simulink model "LQR_SHUM"  (R2015a)
settings: Solver=ode45  StartTime=0.0  StopTime=20  RelTol=1e-3
values from neighbouring files (symbols this model uses):
  Ki = -Kp1(:,1:2)    [Sc_LQR.m]
  Kp = Kp1(:,3:6)    [Sc_LQR.m]
undefined symbols (not defined in the file or in its folder): A, B, C
settings Model: CovSFcnEnable=off  Creator=jordan  LastModifiedBy=Vladislav
settings DebuggingCC: SolverPrmCheckMsg=warning

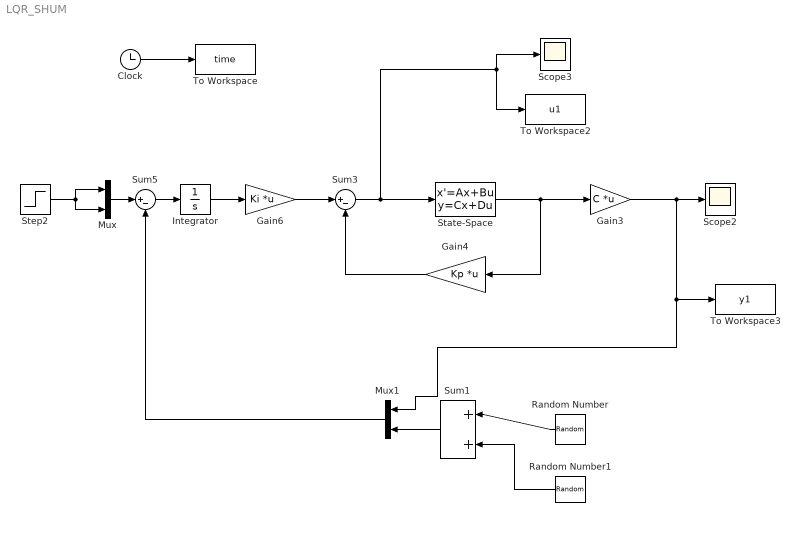
== system LQR_SHUM ==
  Clock : Clock
  Gain3 : Gain  Gain=C  Multiplication=Matrix(K*u)
  Gain4 : Gain  Gain=Kp  Multiplication=Matrix(K*u)
  Gain6 : Gain  Gain=Ki  Multiplication=Matrix(K*u)
  Integrator : Integrator
  Mux : Mux  Inputs=2
  Mux1 : Mux  Inputs=2
  Random Number : RandomNumber  Variance=0.1  SampleTime=0.1
  Random Number1 : RandomNumber  Variance=0.1  Seed=1  SampleTime=0.1
  Scope2 : Scope
      settings: TimeRange=10  YMin=-0.2  YMax=1.4  SaveName=ScopeData2
  Scope3 : Scope
      settings: TimeRange=10  YMin=-0.2  YMax=1.4  SaveName=ScopeData3
  State-Space : StateSpace  A=A  B=B  C=eye(4)  D=zeros(4,2)  X0=0
  Step2 : Step  Time=0  SampleTime=0
  Sum1 : Sum  Inputs=|++
  Sum3 : Sum  Inputs=|+-
  Sum5 : Sum  Inputs=|+-
  To Workspace : ToWorkspace  VariableName=time  SampleTime=-1
  To Workspace2 : ToWorkspace  VariableName=u1  SampleTime=-1
  To Workspace3 : ToWorkspace  VariableName=y1  SampleTime=-1
  wires:
  Sum3/1 -> State-Space/1, To Workspace2/1, Scope3/1
  Gain4/1 -> Sum3/2
  State-Space/1 -> Gain3/1, Gain4/1
  Integrator/1 -> Gain6/1
  Gain6/1 -> Sum3/1
  Step2/1 -> Mux/1, Mux/2
  Mux/1 -> Sum5/1
  Sum5/1 -> Integrator/1
  Gain3/1 -> Mux1/1, To Workspace3/1, Scope2/1
  Clock/1 -> To Workspace/1
  Random Number/1 -> Sum1/1
  Random Number1/1 -> Sum1/2
  Sum1/1 -> Mux1/2
  Mux1/1 -> Sum5/2
